simulink model "logistico"  (R2023b)
settings: Solver=VariableStepAuto  StartTime=0.0  StopTime=10.0  RelTol=1e-3
settings Model: Creator=stefa  LastModifiedBy=stefa

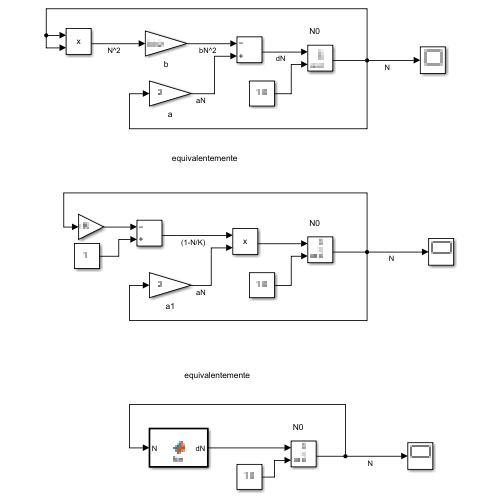
[thumbnail: Simulink's stored preview of the top-level diagram]
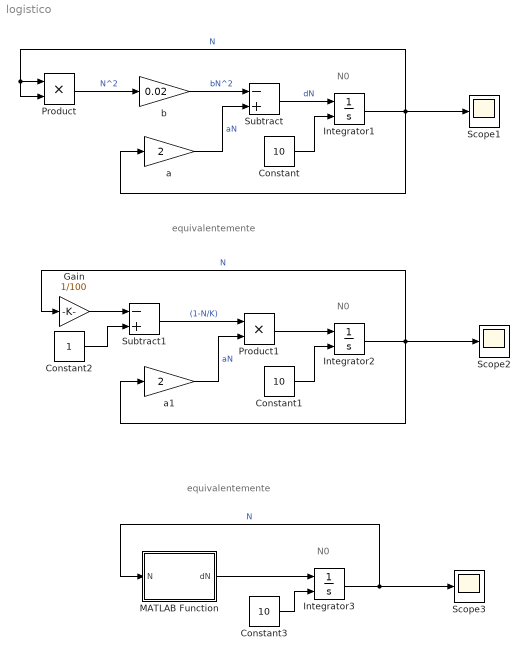
== system logistico ==
  note: equivalentemente
  note: N0
  note: N0
  note: N0
  note: equivalentemente
  Constant : Constant  Value=10
  Constant1 : Constant  Value=10
  Constant2 : Constant
  Constant3 : Constant  Value=10
  Gain : Gain  Gain=1/100
  Integrator1 : Integrator  InitialConditionSource=external  InitialCondition=10
  Integrator2 : Integrator  InitialConditionSource=external  InitialCondition=10
  Integrator3 : Integrator  InitialConditionSource=external  InitialCondition=10
  MATLAB Function : MATLAB Function  TreatAsAtomicUnit=on
  Product : Product
  Product1 : Product
  Scope1 : Scope
  Scope2 : Scope
  Scope3 : Scope
  Subtract : Sum  Inputs=-+
  Subtract1 : Sum  Inputs=-+
  a : Gain  Gain=2
  a1 : Gain  Gain=2
  b : Gain  Gain=0.02
  wires:
  a/1 -> Subtract/2  "aN"
  Integrator1/1 -> Product/2, Product/1, Scope1/1, a/1  "N"
  Subtract/1 -> Integrator1/1  "dN"
  b/1 -> Subtract/1  "bN^2"
  Constant/1 -> Integrator1/2
  Product/1 -> b/1  "N^2"
  Constant1/1 -> Integrator2/2
  Integrator2/1 -> Gain/1, Scope2/1, a1/1  "N"
  a1/1 -> Product1/2  "aN"
  Product1/1 -> Integrator2/1
  Constant2/1 -> Subtract1/2
  Subtract1/1 -> Product1/1  "(1-N/K)"
  Gain/1 -> Subtract1/1
  MATLAB Function/1(dN) -> Integrator3/1
  Integrator3/1 -> MATLAB Function/1(N), Scope3/1  "N"
  Constant3/1 -> Integrator3/2

== matlab function logistico/MATLAB Function ==
  data: N input; dN output
function dN = fcn(N)
a=2;
K=100;
dN=[a*N*(1-N/K)];
